simulink model "DPCvalidation"  (R2021a)
settings: Solver=VariableStepAuto  StartTime=0.0  StopTime=10.0  RelTol=1e-3
undefined symbols (not defined in the file or in its folder): C, errorC, errorL, L, Lc, Lload, Rl, Rload, Ts, Vdc, Vref
libraries: spsIGBTDiodeLib x6, spsThreePhaseSeriesRLCBranchLib x5, spsThreePhaseVIMeasurementLib x3, spsOnDelayLib x3, spsGroundLib x2, spsThreePhaseBreakerLib x2, spsDCVoltageSourceLib x1, deeplib x1, simulink x1
settings Model: Creator=DU47TW  LastModifiedBy=DU47TW

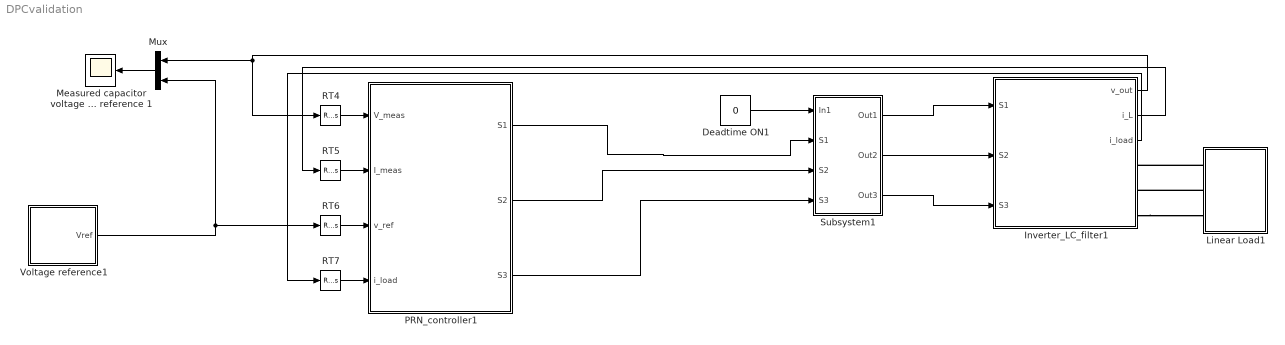
== system DPCvalidation ==
  Deadtime ON1 : Constant  Value=0
  Inverter_LC_filter1 : Subsystem
  Linear Load1 : Subsystem
  Measured capacitor voltage and reference 1 : Scope
  Mux : Mux  Inputs=2
  PRN_controller1 : Subsystem  SystemSampleTime=Ts
  RT{4..7} (4 alike) : RateTransition  OutPortSampleTime=Tsa
  Subsystem1 : Subsystem
  Voltage reference1 : Subsystem
  wires:
  PRN_controller1/1(S1) -> Subsystem1/2(S1)
  Mux/1 -> Measured capacitor voltage and reference 1/1
  Inverter_LC_filter1/2(i_L) -> RT5/1
  Inverter_LC_filter1/1(v_out) -> Mux/1, RT4/1
  PRN_controller1/2(S2) -> Subsystem1/3(S2)
  PRN_controller1/3(S3) -> Subsystem1/4(S3)
  Inverter_LC_filter1/3(i_load) -> RT7/1
  Subsystem1/1(Out1) -> Inverter_LC_filter1/1(S1)
  RT6/1 -> PRN_controller1/3(v_ref)
  RT5/1 -> PRN_controller1/2(I_meas)
  Subsystem1/2(Out2) -> Inverter_LC_filter1/2(S2)
  RT7/1 -> PRN_controller1/4(i_load)
  RT4/1 -> PRN_controller1/1(V_meas)
  Subsystem1/3(Out3) -> Inverter_LC_filter1/3(S3)
  Voltage reference1/1(Vref) -> Mux/2, RT6/1
  Deadtime ON1/1 -> Subsystem1/1(In1)
  connections:
  Linear Load1/LConn2 -- Inverter_LC_filter1/RConn2
  Inverter_LC_filter1/RConn3 -- Linear Load1/LConn3
  Linear Load1/LConn1 -- Inverter_LC_filter1/RConn1

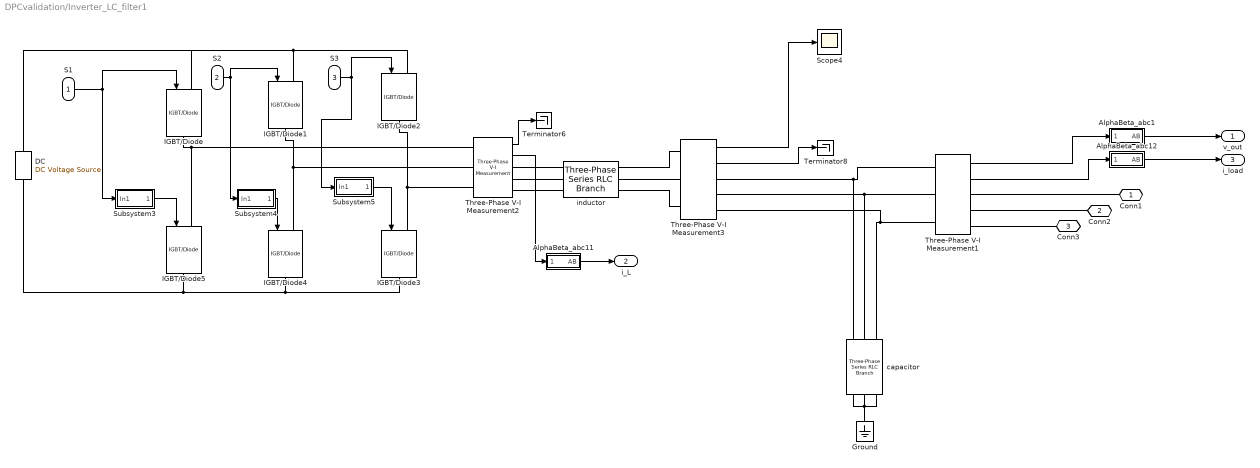
== system DPCvalidation/Inverter_LC_filter1 ==
  S1 : Inport
  S2 : Inport  Port=2
  S3 : Inport  Port=3
  AlphaBeta_abc1 : Subsystem
  AlphaBeta_abc11 : Subsystem
  AlphaBeta_abc12 : Subsystem
  DC : spsDCVoltageSourceLib/DC Voltage Source  Amplitude=Vdc  Measurements=None
  Ground : spsGroundLib/Ground  LConnTagsString=a
  IGBT/Diode{,1..5} (6 alike) : spsIGBTDiodeLib/IGBT//Diode  Ron=1e-3  Rs=1e5  Cs=inf  Measurements=off
  Scope4 : Scope
  Subsystem3 : Subsystem
  Subsystem4 : Subsystem
  Subsystem5 : Subsystem
  Terminator6 : Terminator
  Terminator8 : Terminator
  Three-Phase V-I Measurement1 : spsThreePhaseVIMeasurementLib/Three-Phase V-I Measurement  VoltageMeasurement=phase-to-ground  SetLabelV=off  LabelV=Vabc  Vpu=off  VpuLL=off  CurrentMeasurement=yes  SetLabelI=off  LabelI=Iabc  Ipu=off  Pbase=100e6  Vbase=500e3  OutputType=Complex  PhasorSimulation=off  PSBequivalent=0
  Three-Phase V-I Measurement2 : spsThreePhaseVIMeasurementLib/Three-Phase V-I Measurement  VoltageMeasurement=phase-to-ground  SetLabelV=off  LabelV=Vabc  Vpu=off  VpuLL=off  CurrentMeasurement=yes  SetLabelI=off  LabelI=Iabc  Ipu=off  Pbase=100e6  Vbase=500e3  OutputType=Complex  PhasorSimulation=off  PSBequivalent=0
  Three-Phase V-I Measurement3 : spsThreePhaseVIMeasurementLib/Three-Phase V-I Measurement  VoltageMeasurement=phase-to-ground  SetLabelV=off  LabelV=Vabc  Vpu=off  VpuLL=off  CurrentMeasurement=yes  SetLabelI=off  LabelI=Iabc  Ipu=off  Pbase=100e6  Vbase=500e3  OutputType=Complex  PhasorSimulation=off  PSBequivalent=0
  capacitor : spsThreePhaseSeriesRLCBranchLib/Three-Phase Series RLC Branch  LConnTagsString=A|B|C  RConnTagsString=A|B|C  BranchType=C  Resistance=Rl  Inductance=Lc  Capacitance=C+errorC  Measurements=None
  inductor : spsThreePhaseSeriesRLCBranchLib/Three-Phase Series RLC Branch  LConnTagsString=A|B|C  RConnTagsString=A|B|C  BranchType=RL  Resistance=0  Inductance=L+errorL  Capacitance=1e-6  Measurements=None
  Conn1 : PMIOPort  Side=Right
  Conn2 : PMIOPort  Port=2  Side=Right
  Conn3 : PMIOPort  Port=3  Side=Right
  v_out : Outport  VectorParamsAs1DForOutWhenUnconnected=off
  i_L : Outport  Port=2  VectorParamsAs1DForOutWhenUnconnected=off
  i_load : Outport  Port=3  VectorParamsAs1DForOutWhenUnconnected=off
  wires:
  Three-Phase V-I Measurement2/2 -> AlphaBeta_abc11/1(abc)
  Subsystem5/1(Out1) -> IGBT/Diode3/1
  S2/1 -> IGBT/Diode1/1, Subsystem4/1(In1)
  S1/1 -> IGBT/Diode/1, Subsystem3/1(In1)
  Subsystem4/1(Out1) -> IGBT/Diode4/1
  S3/1 -> IGBT/Diode2/1, Subsystem5/1(In1)
  Subsystem3/1(Out1) -> IGBT/Diode5/1
  AlphaBeta_abc11/1(AB) -> i_L/1
  Three-Phase V-I Measurement1/2 -> AlphaBeta_abc12/1(abc)
  AlphaBeta_abc12/1(AB) -> i_load/1
  Three-Phase V-I Measurement1/1 -> AlphaBeta_abc1/1(abc)
  AlphaBeta_abc1/1(AB) -> v_out/1
  Three-Phase V-I Measurement2/1 -> Terminator6/1
  Three-Phase V-I Measurement3/1 -> Scope4/1
  Three-Phase V-I Measurement3/2 -> Terminator8/1
  connections:
  capacitor/RConn2 -- capacitor/RConn1 -- Ground/LConn1 -- capacitor/RConn3
  Three-Phase V-I Measurement2/RConn1 -- inductor/LConn1
  inductor/LConn2 -- Three-Phase V-I Measurement2/RConn2
  inductor/LConn3 -- Three-Phase V-I Measurement2/RConn3
  IGBT/Diode1/RConn1 -- IGBT/Diode4/LConn1 -- Three-Phase V-I Measurement2/LConn2
  IGBT/Diode2/RConn1 -- Three-Phase V-I Measurement2/LConn3 -- IGBT/Diode3/LConn1
  IGBT/Diode/RConn1 -- IGBT/Diode5/LConn1 -- Three-Phase V-I Measurement2/LConn1
  Three-Phase V-I Measurement1/RConn1 -- Conn1/RConn1
  Three-Phase V-I Measurement1/RConn2 -- Conn2/RConn1
  Three-Phase V-I Measurement1/RConn3 -- Conn3/RConn1
  Three-Phase V-I Measurement3/RConn1 -- Three-Phase V-I Measurement1/LConn1 -- capacitor/LConn1
  Three-Phase V-I Measurement3/RConn2 -- Three-Phase V-I Measurement1/LConn2 -- capacitor/LConn2
  Three-Phase V-I Measurement3/RConn3 -- capacitor/LConn3 -- Three-Phase V-I Measurement1/LConn3
  inductor/RConn2 -- Three-Phase V-I Measurement3/LConn2
  inductor/RConn3 -- Three-Phase V-I Measurement3/LConn3
  inductor/RConn1 -- Three-Phase V-I Measurement3/LConn1
  IGBT/Diode1/LConn1 -- IGBT/Diode/LConn1 -- DC/RConn1 -- IGBT/Diode2/LConn1
  IGBT/Diode5/RConn1 -- DC/LConn1 -- IGBT/Diode3/RConn1 -- IGBT/Diode4/RConn1

== system DPCvalidation/Linear Load1 ==
  Ground3 : spsGroundLib/Ground  LConnTagsString=a
  Linear load : spsThreePhaseSeriesRLCBranchLib/Three-Phase Series RLC Branch  LConnTagsString=A|B|C  RConnTagsString=A|B|C  BranchType=R  Resistance=Rload  Inductance=1e-3  Capacitance=1e-6  Measurements=None
  Linear load1 : spsThreePhaseSeriesRLCBranchLib/Three-Phase Series RLC Branch  LConnTagsString=A|B|C  RConnTagsString=A|B|C  BranchType=R  Resistance=120  Inductance=1e-3  Capacitance=1e-6  Measurements=None
  Linear load2 : spsThreePhaseSeriesRLCBranchLib/Three-Phase Series RLC Branch  LConnTagsString=A|B|C  RConnTagsString=A|B|C  BranchType=R  Resistance=Rload  Inductance=Lload  Capacitance=1e-6  Measurements=None
  Step : Step  Time=0.04  SampleTime=0
  Step1 : Step  Time=0.07  SampleTime=0
  Three-Phase Breaker : spsThreePhaseBreakerLib/Three-Phase Breaker  InitialState=open  SwitchA=on  SwitchB=on  SwitchC=on  SwitchTimes="[1/60  5/60]"  External=on  BreakerResistance=0.01  SnubberResistance=1e6  SnubberCapacitance=inf  Measurements=None
  Three-Phase Breaker1 : spsThreePhaseBreakerLib/Three-Phase Breaker  InitialState=open  SwitchA=on  SwitchB=on  SwitchC=on  SwitchTimes="[1/60  5/60]"  External=on  BreakerResistance=0.01  SnubberResistance=1e6  SnubberCapacitance=inf  Measurements=None
  Conn1 : PMIOPort  Side=Left
  Conn2 : PMIOPort  Port=2  Side=Left
  Conn3 : PMIOPort  Port=3  Side=Left
  wires:
  Step/1 -> Three-Phase Breaker/1
  Step1/1 -> Three-Phase Breaker1/1
  connections:
  Three-Phase Breaker/RConn2 -- Linear load2/LConn2
  Linear load1/RConn2 -- Linear load/RConn2 -- Linear load/RConn1 -- Linear load2/RConn3 -- Linear load2/RConn2 -- Linear load2/RConn1 -- Ground3/LConn1 -- Linear load/RConn3 -- Linear load1/RConn1 -- Linear load1/RConn3
  Three-Phase Breaker/RConn3 -- Linear load2/LConn3
  Three-Phase Breaker/RConn1 -- Linear load2/LConn1
  Conn1/RConn1 -- Three-Phase Breaker/LConn1 -- Linear load/LConn1 -- Three-Phase Breaker1/LConn1
  Conn2/RConn1 -- Three-Phase Breaker/LConn2 -- Linear load/LConn2 -- Three-Phase Breaker1/LConn2
  Conn3/RConn1 -- Three-Phase Breaker/LConn3 -- Linear load/LConn3 -- Three-Phase Breaker1/LConn3
  Linear load1/LConn1 -- Three-Phase Breaker1/RConn1
  Linear load1/LConn2 -- Three-Phase Breaker1/RConn2
  Linear load1/LConn3 -- Three-Phase Breaker1/RConn3

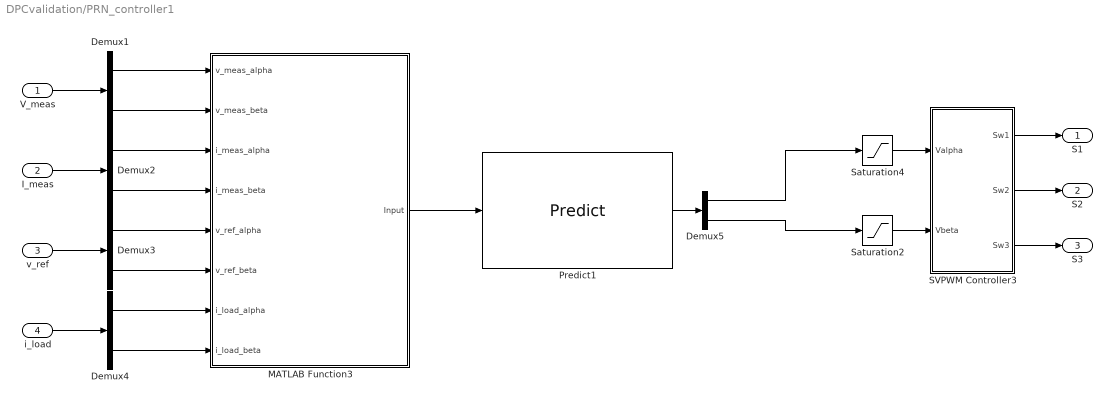
== system DPCvalidation/PRN_controller1 ==
  V_meas : Inport
  I_meas : Inport  Port=2
  v_ref : Inport  Port=3
  i_load : Inport  Port=4
  Demux{1..5} (5 alike) : Demux  Outputs=2
  MATLAB Function3 : MATLAB Function  TreatAsAtomicUnit=on  SystemSampleTime=1e-5
  Predict1 : deeplib/Predict  Network=Network from MAT-file  NetworkFunction=squeezenet  NetworkFilePath=C:\Users\DU47TW\OneDrive - Aalborg Universitet\Desktop\AI Basis\tie-2969116-mm\Supplementary files - new\trainedNet1nDPCv3.mat  MiniBatchSize=128  InputDataFormats={ 'input', 'C' }  Predictions=on  Activations={}  ForceInterpretedSim=off  EnableDLNetwork=on
      settings: SourceProductBaseCode=NN
  SVPWM Controller3 : Subsystem
  Saturation2 : Saturate  UpperLimit=467  LowerLimit=-467
  Saturation4 : Saturate  UpperLimit=467  LowerLimit=-467
  S1 : Outport  VectorParamsAs1DForOutWhenUnconnected=off
  S2 : Outport  Port=2  VectorParamsAs1DForOutWhenUnconnected=off
  S3 : Outport  Port=3  VectorParamsAs1DForOutWhenUnconnected=off
  wires:
  Demux2/2 -> MATLAB Function3/4(i_meas_beta)
  Demux3/2 -> MATLAB Function3/6(v_ref_beta)
  Demux4/1 -> MATLAB Function3/7(i_load_alpha)
  Demux1/1 -> MATLAB Function3/1(v_meas_alpha)
  Demux1/2 -> MATLAB Function3/2(v_meas_beta)
  Demux3/1 -> MATLAB Function3/5(v_ref_alpha)
  Demux2/1 -> MATLAB Function3/3(i_meas_alpha)
  Demux4/2 -> MATLAB Function3/8(i_load_beta)
  I_meas/1 -> Demux2/1
  v_ref/1 -> Demux3/1
  i_load/1 -> Demux4/1
  V_meas/1 -> Demux1/1
  ? -> ?
  SVPWM Controller3/1(Sw1) -> S1/1
  SVPWM Controller3/2(Sw2) -> S2/1
  SVPWM Controller3/3(Sw3) -> S3/1
  Demux5/1 -> Saturation4/1
  Saturation4/1 -> SVPWM Controller3/1(Valpha)
  Demux5/2 -> Saturation2/1
  Saturation2/1 -> SVPWM Controller3/2(Vbeta)
  MATLAB Function3/1(Input) -> Predict1/1
  Predict1/1 -> Demux5/1

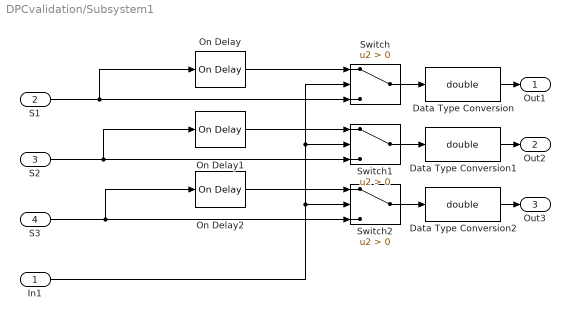
== system DPCvalidation/Subsystem1 ==
  In1 : Inport
  S1 : Inport  Port=2
  S2 : Inport  Port=3
  S3 : Inport  Port=4
  Data Type Conversion : DataTypeConversion  OutDataTypeStr=double
  Data Type Conversion1 : DataTypeConversion  OutDataTypeStr=double
  Data Type Conversion2 : DataTypeConversion  OutDataTypeStr=double
  On Delay : spsOnDelayLib/On Delay  DelayType=On delay  delay=Td  ic=0  Ts=1e-6
      settings: SourceProductBaseCode=PS
  On Delay1 : spsOnDelayLib/On Delay  DelayType=On delay  delay=Td  ic=0  Ts=0
      settings: SourceProductBaseCode=PS
  On Delay2 : spsOnDelayLib/On Delay  DelayType=On delay  delay=Td  ic=0  Ts=0
      settings: SourceProductBaseCode=PS
  Switch : Switch  Criteria=u2 > Threshold
  Switch1 : Switch  Criteria=u2 > Threshold
  Switch2 : Switch  Criteria=u2 > Threshold
  Out1 : Outport
  Out2 : Outport  Port=2
  Out3 : Outport  Port=3
  wires:
  In1/1 -> Switch/2, Switch1/2, Switch2/2
  On Delay/1 -> Switch/1
  S3/1 -> On Delay2/1, Switch2/3
  On Delay1/1 -> Switch1/1
  S2/1 -> On Delay1/1, Switch1/3
  Switch2/1 -> Data Type Conversion2/1
  S1/1 -> Switch/3, On Delay/1
  On Delay2/1 -> Switch2/1
  Switch/1 -> Data Type Conversion/1
  Switch1/1 -> Data Type Conversion1/1
  Data Type Conversion/1 -> Out1/1
  Data Type Conversion1/1 -> Out2/1
  Data Type Conversion2/1 -> Out3/1

== system DPCvalidation/Voltage reference1 ==
  AlphaBeta_abc11 : Subsystem
  Mux12 : Mux  Inputs=3
  Voltage_reference_creator : Subsystem
  freq : Gain  Gain=50
  gain : Constant  Value=2*pi
  Vref : Outport  VectorParamsAs1DForOutWhenUnconnected=off
  wires:
  Voltage_reference_creator/1(va*) -> Mux12/1
  AlphaBeta_abc11/1(AB) -> Vref/1
  Voltage_reference_creator/2(vb*) -> Mux12/2
  gain/1 -> freq/1
  Voltage_reference_creator/3(vc*) -> Mux12/3
  Mux12/1 -> AlphaBeta_abc11/1(abc)
  freq/1 -> Voltage_reference_creator/1(wref)

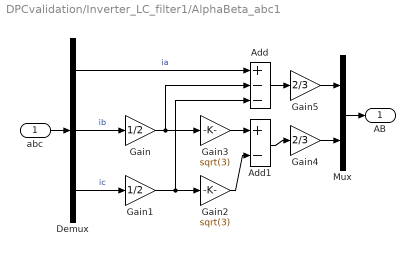
== system DPCvalidation/Inverter_LC_filter1/AlphaBeta_abc1 ==
  abc : Inport
  Add : Sum  Inputs=+--
  Add1 : Sum  Inputs=+-
  Demux : Demux  Outputs=3
  Gain : Gain  Gain=1/2
  Gain1 : Gain  Gain=1/2
  Gain2 : Gain  Gain=sqrt(3)
  Gain3 : Gain  Gain=sqrt(3)
  Gain4 : Gain  Gain=2/3
  Gain5 : Gain  Gain=2/3
  Mux : Mux  Inputs=2
  AB : Outport  VectorParamsAs1DForOutWhenUnconnected=off
  wires:
  abc/1 -> Demux/1
  Gain/1 -> Gain3/1, Add/2
  Gain1/1 -> Gain2/1, Add/3
  Add1/1 -> Gain4/1
  Mux/1 -> AB/1
  Gain3/1 -> Add1/1
  Gain2/1 -> Add1/2
  Add/1 -> Gain5/1
  Demux/1 -> Add/1  "ia"
  Demux/2 -> Gain/1  "ib"
  Demux/3 -> Gain1/1  "ic"
  Gain5/1 -> Mux/1
  Gain4/1 -> Mux/2

== system DPCvalidation/Inverter_LC_filter1/AlphaBeta_abc11 ==
  abc : Inport
  Add : Sum  Inputs=+--
  Add1 : Sum  Inputs=+-
  Demux : Demux  Outputs=3
  Gain : Gain  Gain=1/2
  Gain1 : Gain  Gain=1/2
  Gain2 : Gain  Gain=sqrt(3)
  Gain3 : Gain  Gain=sqrt(3)
  Gain4 : Gain  Gain=2/3
  Gain5 : Gain  Gain=2/3
  Mux : Mux  Inputs=2
  AB : Outport  VectorParamsAs1DForOutWhenUnconnected=off
  wires:
  abc/1 -> Demux/1
  Gain/1 -> Gain3/1, Add/2
  Gain1/1 -> Gain2/1, Add/3
  Add1/1 -> Gain4/1
  Mux/1 -> AB/1
  Gain3/1 -> Add1/1
  Gain2/1 -> Add1/2
  Add/1 -> Gain5/1
  Demux/1 -> Add/1  "ia"
  Demux/2 -> Gain/1  "ib"
  Demux/3 -> Gain1/1  "ic"
  Gain5/1 -> Mux/1
  Gain4/1 -> Mux/2

== system DPCvalidation/Inverter_LC_filter1/AlphaBeta_abc12 ==
  abc : Inport
  Add : Sum  Inputs=+--
  Add1 : Sum  Inputs=+-
  Demux : Demux  Outputs=3
  Gain : Gain  Gain=1/2
  Gain1 : Gain  Gain=1/2
  Gain2 : Gain  Gain=sqrt(3)
  Gain3 : Gain  Gain=sqrt(3)
  Gain4 : Gain  Gain=2/3
  Gain5 : Gain  Gain=2/3
  Mux : Mux  Inputs=2
  AB : Outport  VectorParamsAs1DForOutWhenUnconnected=off
  wires:
  Gain4/1 -> Mux/2
  Gain5/1 -> Mux/1
  Demux/3 -> Gain1/1  "ic"
  Demux/2 -> Gain/1  "ib"
  Demux/1 -> Add/1  "ia"
  Add/1 -> Gain5/1
  Gain2/1 -> Add1/2
  Gain3/1 -> Add1/1
  Mux/1 -> AB/1
  Add1/1 -> Gain4/1
  Gain1/1 -> Add/3, Gain2/1
  Gain/1 -> Add/2, Gain3/1
  abc/1 -> Demux/1

== system DPCvalidation/Inverter_LC_filter1/Subsystem3 ==
  In1 : Inport
  Abs : Abs
  Add : Sum  Inputs=+-
  Constant : Constant
  Out1 : Outport  VectorParamsAs1DForOutWhenUnconnected=off
  wires:
  Constant/1 -> Add/2
  Abs/1 -> Out1/1
  In1/1 -> Add/1
  Add/1 -> Abs/1

== system DPCvalidation/Inverter_LC_filter1/Subsystem4 ==
  In1 : Inport
  Abs : Abs
  Add : Sum  Inputs=+-
  Constant : Constant
  Out1 : Outport  VectorParamsAs1DForOutWhenUnconnected=off
  wires:
  Add/1 -> Abs/1
  In1/1 -> Add/1
  Abs/1 -> Out1/1
  Constant/1 -> Add/2

== system DPCvalidation/Inverter_LC_filter1/Subsystem5 ==
  In1 : Inport
  Abs : Abs
  Add : Sum  Inputs=+-
  Constant : Constant
  Out1 : Outport  VectorParamsAs1DForOutWhenUnconnected=off
  wires:
  Constant/1 -> Add/2
  Abs/1 -> Out1/1
  In1/1 -> Add/1
  Add/1 -> Abs/1

== system DPCvalidation/PRN_controller1/SVPWM Controller3 ==
  Valpha : Inport
  Vbeta : Inport  Port=2
  Subsystem : Subsystem
  Sw1 : Outport  VectorParamsAs1DForOutWhenUnconnected=off
  Sw2 : Outport  Port=2  VectorParamsAs1DForOutWhenUnconnected=off
  Sw3 : Outport  Port=3  VectorParamsAs1DForOutWhenUnconnected=off
  wires:
  Vbeta/1 -> Subsystem/2(Ubeta)
  Valpha/1 -> Subsystem/1(Ualpha)
  Subsystem/3(Sc) -> Sw3/1
  Subsystem/2(Sb) -> Sw2/1
  Subsystem/1(Sa) -> Sw1/1

== system DPCvalidation/Voltage reference1/AlphaBeta_abc11 ==
  abc : Inport
  Add : Sum  Inputs=+--
  Add1 : Sum  Inputs=+-
  Demux : Demux  Outputs=3
  Gain : Gain  Gain=1/2
  Gain1 : Gain  Gain=1/2
  Gain2 : Gain  Gain=sqrt(3)
  Gain3 : Gain  Gain=sqrt(3)
  Gain4 : Gain  Gain=2/3
  Gain5 : Gain  Gain=2/3
  Mux : Mux  Inputs=2
  AB : Outport  VectorParamsAs1DForOutWhenUnconnected=off
  wires:
  abc/1 -> Demux/1
  Gain/1 -> Gain3/1, Add/2
  Gain1/1 -> Gain2/1, Add/3
  Add1/1 -> Gain4/1
  Mux/1 -> AB/1
  Gain3/1 -> Add1/1
  Gain2/1 -> Add1/2
  Add/1 -> Gain5/1
  Demux/1 -> Add/1  "ia"
  Demux/2 -> Gain/1  "ib"
  Demux/3 -> Gain1/1  "ic"
  Gain5/1 -> Mux/1
  Gain4/1 -> Mux/2

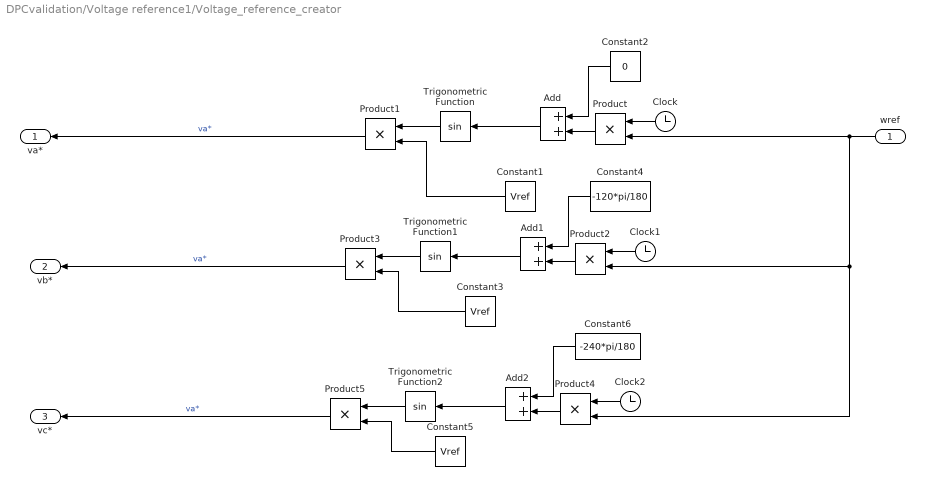
== system DPCvalidation/Voltage reference1/Voltage_reference_creator ==
  wref : Inport
  Add : Sum
  Add1 : Sum
  Add2 : Sum
  Clock : Clock
  Clock1 : Clock
  Clock2 : Clock
  Constant1 : Constant  Value=Vref
  Constant2 : Constant  Value=0
  Constant3 : Constant  Value=Vref
  Constant4 : Constant  Value=-120*pi/180
  Constant5 : Constant  Value=Vref
  Constant6 : Constant  Value=-240*pi/180
  Product{,1..5} (6 alike) : Product
  Trigonometric Function : Trigonometry
  Trigonometric Function1 : Trigonometry
  Trigonometric Function2 : Trigonometry
  va* : Outport  VectorParamsAs1DForOutWhenUnconnected=off
  vb* : Outport  Port=2  VectorParamsAs1DForOutWhenUnconnected=off
  vc* : Outport  Port=3  VectorParamsAs1DForOutWhenUnconnected=off
  wires:
  Product1/1 -> va*/1  "va*"
  Add/1 -> Trigonometric Function/1
  Constant2/1 -> Add/1
  wref/1 -> Product/2, Product2/2, Product4/2
  Trigonometric Function/1 -> Product1/1
  Product/1 -> Add/2
  Clock/1 -> Product/1
  Product3/1 -> vb*/1  "va*"
  Add1/1 -> Trigonometric Function1/1
  Constant4/1 -> Add1/1
  Trigonometric Function1/1 -> Product3/1
  Product2/1 -> Add1/2
  Clock1/1 -> Product2/1
  Product5/1 -> vc*/1  "va*"
  Add2/1 -> Trigonometric Function2/1
  Constant6/1 -> Add2/1
  Trigonometric Function2/1 -> Product5/1
  Product4/1 -> Add2/2
  Clock2/1 -> Product4/1
  Constant1/1 -> Product1/2
  Constant3/1 -> Product3/2
  Constant5/1 -> Product5/2

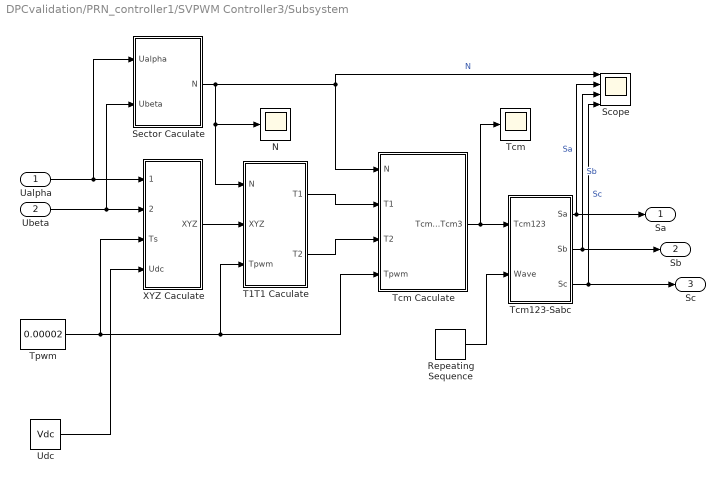
== system DPCvalidation/PRN_controller1/SVPWM Controller3/Subsystem ==
  Ualpha : Inport
  Ubeta : Inport  Port=2
  N : Scope
  Repeating Sequence : simulink/Sources/Repeating Sequence  rep_seq_t=[0 1/100000 1/50000]  rep_seq_y=[0 1/100000 0]
  Scope : Scope  NumInputPorts=4
  Sector Caculate : Subsystem
  T1T1 Caculate : Subsystem
  Tcm : Scope
  Tcm Caculate : Subsystem
  Tcm123-Sabc : Subsystem
  Tpwm : Constant  Value=0.00002
  Udc : Constant  Value=Vdc
  XYZ Caculate : Subsystem
  Sa : Outport
  Sb : Outport  Port=2
  Sc : Outport  Port=3
  wires:
  Ubeta/1 -> XYZ Caculate/2(Ubeta), Sector Caculate/2(Ubeta)
  Ualpha/1 -> Sector Caculate/1(Ualpha), XYZ Caculate/1(Ualpha)
  Tcm123-Sabc/1(Sa) -> Scope/2, Sa/1  "Sa"
  Repeating Sequence/1 -> Tcm123-Sabc/2(Wave)
  Tcm123-Sabc/3(Sc) -> Scope/4, Sc/1  "Sc"
  XYZ Caculate/1(XYZ) -> T1T1 Caculate/2(XYZ)
  T1T1 Caculate/1(T1) -> Tcm Caculate/2(T1)
  Tcm123-Sabc/2(Sb) -> Scope/3, Sb/1  "Sb"
  Tpwm/1 -> XYZ Caculate/3(Ts), T1T1 Caculate/3(Tpwm), Tcm Caculate/4(Tpwm)
  Sector Caculate/1("N ") -> T1T1 Caculate/1(N), N/1, Tcm Caculate/1(N), Scope/1  "N"
  Udc/1 -> XYZ Caculate/4(Udc)
  T1T1 Caculate/2(T2) -> Tcm Caculate/3(T2)
  Tcm Caculate/1(Tcm1 Tcm2 Tcm3) -> Tcm/1, Tcm123-Sabc/1(Tcm123)

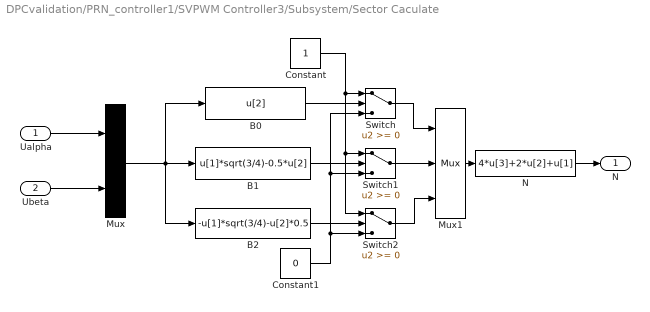
== system DPCvalidation/PRN_controller1/SVPWM Controller3/Subsystem/Sector Caculate ==
  Ualpha : Inport
  Ubeta : Inport  Port=2
  B0 : Fcn  Expr=u[2]
  B1 : Fcn  Expr=u[1]*sqrt(3/4)-0.5*u[2]
  B2 : Fcn  Expr=-u[1]*sqrt(3/4)-u[2]*0.5
  Constant : Constant
  Constant1 : Constant  Value=0
  Mux : Mux  Inputs=2
  Mux1 : Mux  Inputs=3
  N : Fcn  Expr=4*u[3]+2*u[2]+u[1]
  Switch : Switch
  Switch1 : Switch
  Switch2 : Switch
  "N " : Outport
  wires:
  N/1 -> "N "/1
  Mux1/1 -> N/1
  Switch1/1 -> Mux1/2
  Constant1/1 -> Switch2/3, Switch1/3, Switch/3
  Constant/1 -> Switch1/1, Switch2/1, Switch/1
  B2/1 -> Switch2/2
  B1/1 -> Switch1/2
  B0/1 -> Switch/2
  Mux/1 -> B0/1, B1/1, B2/1
  Ubeta/1 -> Mux/2
  Ualpha/1 -> Mux/1
  Switch/1 -> Mux1/1
  Switch2/1 -> Mux1/3

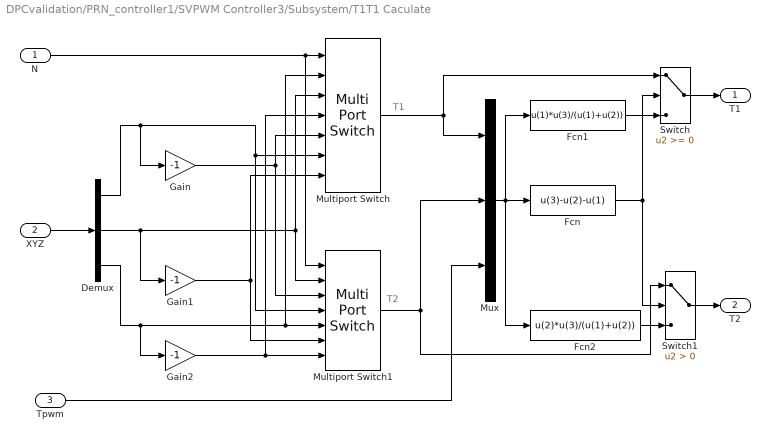
== system DPCvalidation/PRN_controller1/SVPWM Controller3/Subsystem/T1T1 Caculate ==
  note: T2
  note: T1
  N : Inport
  XYZ : Inport  Port=2
  Tpwm : Inport  Port=3
  Demux : Demux  Outputs=3
  Fcn : Fcn  Expr=u(3)-u(2)-u(1)
  Fcn1 : Fcn  Expr=u(1)*u(3)/(u(1)+u(2))
  Fcn2 : Fcn  Expr=u(2)*u(3)/(u(1)+u(2))
  Gain : Gain  Gain=-1
  Gain1 : Gain  Gain=-1
  Gain2 : Gain  Gain=-1
  Multiport Switch : MultiPortSwitch  Inputs=6
  Multiport Switch1 : MultiPortSwitch  Inputs=6
  Mux : Mux  Inputs=3
  Switch : Switch
  Switch1 : Switch  Criteria=u2 > Threshold
  T1 : Outport
  T2 : Outport  Port=2
  wires:
  Gain1/1 -> Multiport Switch/7, Multiport Switch1/6
  Gain2/1 -> Multiport Switch1/7, Multiport Switch/4
  Gain/1 -> Multiport Switch/5, Multiport Switch1/3
  Demux/1 -> Gain/1, Multiport Switch1/4, Multiport Switch/6
  Demux/3 -> Gain2/1, Multiport Switch/2, Multiport Switch1/5
  Demux/2 -> Gain1/1, Multiport Switch1/2, Multiport Switch/3
  N/1 -> Multiport Switch1/1, Multiport Switch/1
  Multiport Switch1/1 -> Mux/2, Switch1/1
  Multiport Switch/1 -> Mux/1, Switch/1
  Mux/1 -> Fcn2/1, Fcn/1, Fcn1/1
  Fcn/1 -> Switch1/2, Switch/2
  Fcn1/1 -> Switch/3
  Fcn2/1 -> Switch1/3
  Switch/1 -> T1/1
  Switch1/1 -> T2/1
  XYZ/1 -> Demux/1
  Tpwm/1 -> Mux/3

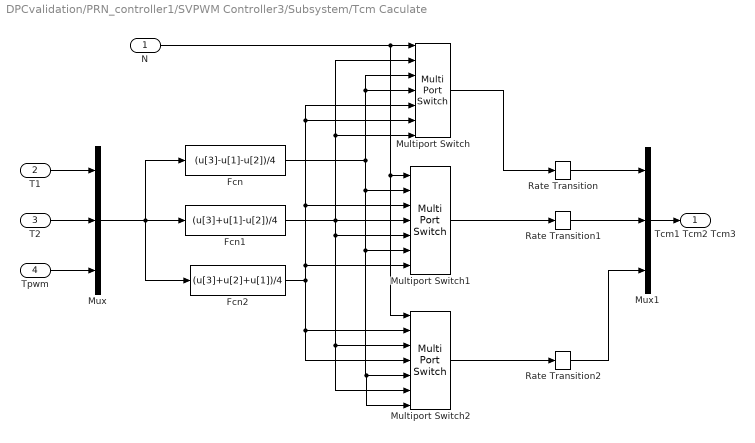
== system DPCvalidation/PRN_controller1/SVPWM Controller3/Subsystem/Tcm Caculate ==
  N : Inport
  T1 : Inport  Port=2
  T2 : Inport  Port=3
  Tpwm : Inport  Port=4
  Fcn : Fcn  Expr=(u[3]-u[1]-u[2])/4
  Fcn1 : Fcn  Expr=(u[3]+u[1]-u[2])/4
  Fcn2 : Fcn  Expr=(u[3]+u[2]+u[1])/4
  Multiport Switch : MultiPortSwitch  Inputs=6
  Multiport Switch1 : MultiPortSwitch  Inputs=6
  Multiport Switch2 : MultiPortSwitch  Inputs=6
  Mux : Mux  Inputs=3
  Mux1 : Mux  Inputs=3
  Rate Transition : RateTransition  OutPortSampleTime=2e-6
  Rate Transition1 : RateTransition  OutPortSampleTime=2e-6
  Rate Transition2 : RateTransition  OutPortSampleTime=2e-6
  Tcm1 Tcm2 Tcm3 : Outport
  wires:
  Rate Transition2/1 -> Mux1/3
  Rate Transition/1 -> Mux1/1
  Multiport Switch2/1 -> Rate Transition2/1
  Multiport Switch1/1 -> Rate Transition1/1
  Rate Transition1/1 -> Mux1/2
  Multiport Switch/1 -> Rate Transition/1
  N/1 -> Multiport Switch/1, Multiport Switch1/1, Multiport Switch2/1
  Fcn2/1 -> Multiport Switch2/4, Multiport Switch2/2, Multiport Switch1/7, Multiport Switch1/3, Multiport Switch/6, Multiport Switch/5
  Fcn1/1 -> Multiport Switch/2, Multiport Switch/7, Multiport Switch1/4, Multiport Switch2/6, Multiport Switch2/3, Multiport Switch1/5
  Fcn/1 -> Multiport Switch1/2, Multiport Switch2/7, Multiport Switch2/5, Multiport Switch1/6, Multiport Switch/4, Multiport Switch/3
  Mux1/1 -> Tcm1 Tcm2 Tcm3/1
  T1/1 -> Mux/1
  T2/1 -> Mux/2
  Tpwm/1 -> Mux/3
  Mux/1 -> Fcn1/1, Fcn/1, Fcn2/1

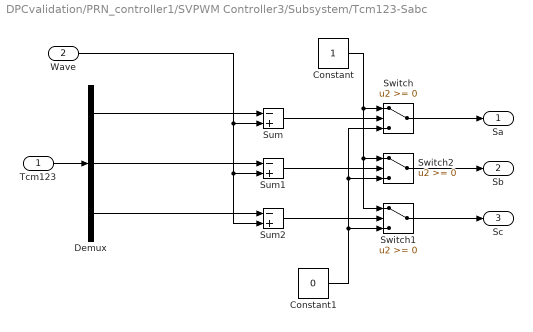
== system DPCvalidation/PRN_controller1/SVPWM Controller3/Subsystem/Tcm123-Sabc ==
  Tcm123 : Inport
  Wave : Inport  Port=2
  Constant : Constant
  Constant1 : Constant  Value=0
  Demux : Demux  Outputs=3
  Sum : Sum  Inputs=-+  SaturateOnIntegerOverflow=on
  Sum1 : Sum  Inputs=-+  SaturateOnIntegerOverflow=on
  Sum2 : Sum  Inputs=-+  SaturateOnIntegerOverflow=on
  Switch : Switch  SaturateOnIntegerOverflow=on
  Switch1 : Switch  SaturateOnIntegerOverflow=on
  Switch2 : Switch  SaturateOnIntegerOverflow=on
  Sa : Outport
  Sb : Outport  Port=2
  Sc : Outport  Port=3
  wires:
  Wave/1 -> Sum/2, Sum2/2, Sum1/2
  Demux/1 -> Sum/1
  Demux/2 -> Sum1/1
  Demux/3 -> Sum2/1
  Tcm123/1 -> Demux/1
  Sum/1 -> Switch/2
  Sum1/1 -> Switch2/2
  Sum2/1 -> Switch1/2
  Constant/1 -> Switch1/1, Switch2/1, Switch/1
  Constant1/1 -> Switch/3, Switch2/3, Switch1/3
  Switch/1 -> Sa/1
  Switch2/1 -> Sb/1
  Switch1/1 -> Sc/1

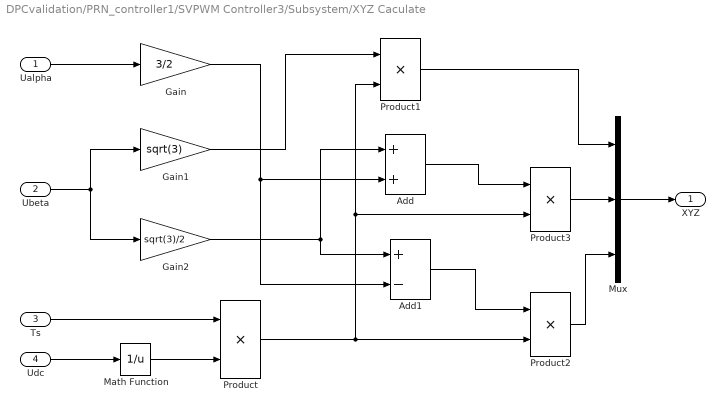
== system DPCvalidation/PRN_controller1/SVPWM Controller3/Subsystem/XYZ Caculate ==
  Ualpha : Inport
  Ubeta : Inport  Port=2
  Ts : Inport  Port=3
  Udc : Inport  Port=4
  Add : Sum
  Add1 : Sum  Inputs=+-
  Gain : Gain  Gain=3/2
  Gain1 : Gain  Gain=sqrt(3)
  Gain2 : Gain  Gain=sqrt(3)/2
  Math Function : Math  Operator=reciprocal  SignedPower=on  SaturateOnIntegerOverflow=on
  Mux : Mux  Inputs=3
  Product{,1..3} (4 alike) : Product  RndMeth=Zero
  XYZ : Outport
  wires:
  Add/1 -> Product3/1
  Add1/1 -> Product2/1
  Gain2/1 -> Add1/1, Add/1
  Gain/1 -> Add/2, Add1/2
  Product/1 -> Product3/2, Product1/2, Product2/2
  Gain1/1 -> Product1/1
  Ts/1 -> Product/1
  Math Function/1 -> Product/2
  Udc/1 -> Math Function/1
  Ubeta/1 -> Gain1/1, Gain2/1
  Ualpha/1 -> Gain/1
  Product2/1 -> Mux/3
  Product3/1 -> Mux/2
  Product1/1 -> Mux/1
  Mux/1 -> XYZ/1

== matlab function DPCvalidation/PRN_controller1/MATLAB Function3 ==
  data: v_meas_alpha input; Input output; v_meas_beta input; i_meas_alpha input; i_meas_beta input; v_ref_alpha input; v_ref_beta input; i_load_alpha input; i_load_beta input
function Input = mes(v_meas_alpha,v_meas_beta, i_meas_alpha,i_meas_beta, v_ref_alpha, v_ref_beta, i_load_alpha, i_load_beta)

Input = zeros(1, 7); 

R1 = sqrt(v_meas_alpha^2 + v_meas_beta^2) / sqrt(i_load_alpha^2 + i_load_beta^2);



Input=[i_meas_alpha,i_meas_beta,v_meas_alpha,v_meas_beta,v_ref_alpha,v_ref_beta,R1];
